simulink model "AM_Modulator_and_Demodulator"  (R2021a)
settings: Solver=VariableStepAuto  StartTime=0.0  StopTime=2  RelTol=1e-3
libraries: dspfdesign x3
settings Model: Creator=ZephyrY  LastModifiedBy=ZephyrY

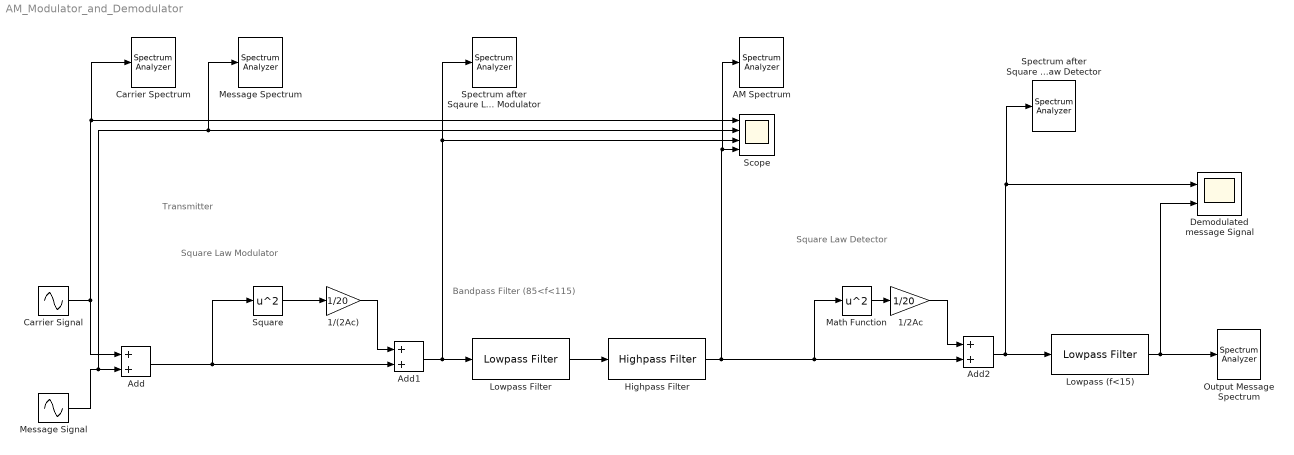
== system AM_Modulator_and_Demodulator ==
  note: Transmitter
  note: Square Law Detector
  note: Bandpass Filter (85<f<115)
  note: Square Law Modulator
  1/(2Ac) : Gain  Gain=1/20
  1/2Ac : Gain  Gain=1/20
  AM Spectrum : SpectrumAnalyzer
  Add : Sum
  Add1 : Sum
  Add2 : Sum
  Carrier Signal : Sin  Amplitude=10  Frequency=2*pi*100  Phase=pi/2  SampleTime=1e-3
  Carrier Spectrum : SpectrumAnalyzer
  Demodulated message Signal : Scope  NumInputPorts=2
  Highpass Filter : dspfdesign/Highpass Filter  FilterType=FIR  DesignForMinimumOrder=off  FilterOrder=50  StopbandFrequency=8e3  PassbandFrequency=85  StopbandAttenuation=80  PassbandRipple=0.1  InheritSampleRate=on  SampleRate=44100  SimulateUsing=Interpreted execution  roundingMode=Floor  coeffsDataTypeStr=fixdt(1,16)
  Lowpass (f<15) : dspfdesign/Lowpass Filter  FilterType=FIR  DesignForMinimumOrder=off  FilterOrder=200  PassbandFrequency=11  StopbandFrequency=12e3  PassbandRipple=0.1  StopbandAttenuation=80  InheritSampleRate=on  SampleRate=44100  SimulateUsing=Interpreted execution  roundingMode=Floor  coeffsDataTypeStr=fixdt(1,16)
  Lowpass Filter : dspfdesign/Lowpass Filter  FilterType=FIR  DesignForMinimumOrder=off  FilterOrder=50  PassbandFrequency=115  StopbandFrequency=12e3  PassbandRipple=0.1  StopbandAttenuation=80  InheritSampleRate=on  SampleRate=44100  SimulateUsing=Interpreted execution  roundingMode=Floor  coeffsDataTypeStr=fixdt(1,16)
  Math Function : Math  Operator=square  SaturateOnIntegerOverflow=on
  Message Signal : Sin  Amplitude=5  Frequency=2*pi*10  Phase=pi/2  SampleTime=1e-3
  Message Spectrum : SpectrumAnalyzer
  Output Message Spectrum : SpectrumAnalyzer
  Scope : Scope  NumInputPorts=4
  Spectrum after Square Law Detector : SpectrumAnalyzer
  Spectrum after Sqaure Law Modulator : SpectrumAnalyzer
  Square : Math  Operator=square  SaturateOnIntegerOverflow=on
  wires:
  Carrier Signal/1 -> Add/1, Carrier Spectrum/1, Scope/1
  Message Signal/1 -> Message Spectrum/1, Scope/2, Add/2
  Add/1 -> Add1/2, Square/1
  Square/1 -> 1/(2Ac)/1
  1/(2Ac)/1 -> Add1/1
  Add1/1 -> Spectrum after Sqaure Law Modulator/1, Scope/3, Lowpass Filter/1
  Lowpass Filter/1 -> Highpass Filter/1
  Highpass Filter/1 -> AM Spectrum/1, Scope/4, Add2/2, Math Function/1
  Math Function/1 -> 1/2Ac/1
  1/2Ac/1 -> Add2/1
  Add2/1 -> Spectrum after Square Law Detector/1, Demodulated message Signal/1, Lowpass (f<15)/1
  Lowpass (f<15)/1 -> Output Message Spectrum/1, Demodulated message Signal/2
